simulink model "AndBroadcast_2018a"  (R2018a)
settings: Solver=VariableStepAuto  StartTime=0.0  StopTime=10.0  RelTol=1e-3
settings Model: Creator=apple  LastModifiedBy=apple
settings DataIOCC: ReturnWorkspaceOutputs=on
settings SFSimCC: SimUseLocalCustomCode=on
settings RTWCC: RTWUseLocalCustomCode=on

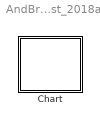
== system AndBroadcast_2018a ==
  Chart : Stateflow chart  TreatAsAtomicUnit=on

== stateflow chart AndBroadcast_2018a/Chart ==
  state A
    en:fprintf("Entry A");
    du:fprintf("During A");
    ex:fprintf("Exit A");
    state A1 [parallel]
      en:fprintf("Entry A1");
      du:fprintf("During A1");
      ex:fprintf("Exit A1");
      settings: executionOrder=1
      state A1a
        en:fprintf("Entry A1a");
        du:fprintf("During A1a");
        ex:fprintf("Exit A1a");
      state A1b
        en:fprintf("Entry A1b");
        du:fprintf("During A1b");
        ex:fprintf("Exit A1b");
      (default) -> A1a
      A1a -> A.A1.A1b : E_one{send(E_two)}
    state A2 [parallel]
      en:fprintf("Entry A2");
      du:fprintf("During A2");
      ex:fprintf("Exit A2");
      settings: executionOrder=2
      state A2a
        en:fprintf("Entry A2a");
        du:fprintf("During A2a");
        ex:fprintf("Exit A2a");
      state A1b
        en:fprintf("Entry A2b");
        du:fprintf("During A2b");
        ex:fprintf("Exit A2b");
      (default) -> A2a
      A2a -> A.A2.A1b : E_two
  (default) -> A
  events: E_one local FUNCTION_CALL_EVENT; E_two local FUNCTION_CALL_EVENT
